simulink model "MPC"  (R2024b)
settings: Solver=ode4  StartTime=0.0  StopTime=tsim  FixedStep=baseRate  RelTol=1e-6  AbsTol=1e-6
values from neighbouring files (symbols this model uses):
  C = [cos(theta), -sin(theta) ... (first row only)    [Run_Initializer.m]    (also in plotBatch.m = quat2Rotm(q','scalarFirst'))
  camera_FOV = 40*d2r    (= 0.698131700798)    [Run_Initializer.m]
  camera_offset = [0.145, 0.087]'    [Run_Initializer.m]
  docking_face = [0 1]'    [Run_Initializer.m]
  docking_offset = [0 0 0]'    [Run_Initializer.m]
  eta = 0.7    [Run_Initializer.m]
  F_t = [kron(eye(N_h),  [zeros(2,3), eye(2), zeros(2,4)]) ... (first row only)    [Run_Initializer.m]
  f_t = [kron(ones(N_h, 1), [xLength yLength]' - edge_buffer) ... (first row only)    [Run_Initializer.m]
  F_u = [kron(eye(N_h),  [eye(3), zeros(3,6)]) ... (first row only)    [Run_Initializer.m]
  f_u = kron(ones(2*N_h, 1), u_max')    [Run_Initializer.m]
  F_v = [kron(eye(N_h),  [zeros(1,5), 1, zeros(1,3)]) ... (first row only)    [Run_Initializer.m]
  gamma = 0.95    [Run_Initializer.m]
  Gamma1_el = 0.12    [Run_Initializer.m]
  Gamma1_sh = 0.005    [Run_Initializer.m]
  Gamma1_wr = 0.025    [Run_Initializer.m]
  Gamma2_el = 5    [Run_Initializer.m]
  Gamma2_sh = 5    [Run_Initializer.m]
  Gamma2_wr = 5    [Run_Initializer.m]
  Gamma3_el = 10    [Run_Initializer.m]
  Gamma3_sh = 40    [Run_Initializer.m]
  Gamma3_wr = 40    [Run_Initializer.m]
  Gamma4_el = 0.039    [Run_Initializer.m]
  Gamma4_sh = 0.015    [Run_Initializer.m]
  Gamma4_wr = 0.029    [Run_Initializer.m]
  Gamma5_el = 800    [Run_Initializer.m]
  Gamma5_sh = 800    [Run_Initializer.m]
  Gamma5_wr = 800    [Run_Initializer.m]
  Gamma6_el = 0.000001    (= 1e-06)    [Run_Initializer.m]
  Gamma6_sh = 0.005    [Run_Initializer.m]
  Gamma6_wr = 0.02    [Run_Initializer.m]
  H = kron(eye(N_h), [R, zeros(3,6); zeros(6,3), Q])    [Run_Initializer.m]
  IBLACK = 0.1996    [unpackData.m]
  IRED = 0.1982    [unpackData.m]
  J = sum(wp*posErr + wt*angErr)    [find_transformation.m]
  Kd_elarm = 0.8    [Run_Initializer.m]
  Kd_sharm = 1.0    (= 1)    [Run_Initializer.m]
  Kd_wrarm = 0.6    [Run_Initializer.m]
  Kp_elarm = 1.2    [Run_Initializer.m]
  Kp_sharm = 1.5    [Run_Initializer.m]
  Kp_wrarm = 1.0    (= 1)    [Run_Initializer.m]
  m = m + 5    (= 4)    [unpackData.m]
  M = diag([1/m; 1/m; 1/I])    [unpackData.m]
  maxd = [d1 ... (first row only)    [Run_Initializer.m]
  mBLACK = 11.3620    (= 11.362)    [unpackData.m]
  mRED = 11.2970    (= 11.297)    [unpackData.m]
  N = size(rel,1)    [plotBatch.m]    (also in unpackData.m = 0)
  p = [0 obj.pos(k,:)]    [SparseState6DOF.m]
  PDQ = blkdiag(20*eye(3),eye(3), 20*eye(3),eye(3))    [Run_Initializer.m]
  PQ = blkdiag(20*eye(6),eye(6))    [Run_Initializer.m]
  PR = blkdiag(20*eye(3), eye(6), 0.0001*eye(3))    [Run_Initializer.m]
  PWMFreq = 5    [Run_Initializer.m]
  Q = diag([100 100 100 300 300 300])    [Run_Initializer.m]    (also in unpackData.m = blkdiag(0.0001*eye(2), 0.00001))
  R = diag([200 200 200])    [Run_Initializer.m]    (also in plotBatch.m = C3(yaw); unpackData.m = diag([6;6;6]))
  r_hold_obs = 1.1*sqrt(2)*0.3.*[1 1]    [Run_Initializer.m]
  r_hold_tar_min = [0.8; (0.3+0.05)]    [Run_Initializer.m]
  rho = 0.98    [Run_Initializer.m]
  T_d = 2    [Run_Initializer.m]
  T_max = 0.15    [Run_Initializer.m]
  Tz_lim_elarm = .1    (= 0.1)    [Run_Initializer.m]
  Tz_lim_sharm = .1    (= 0.1)    [Run_Initializer.m]
  Tz_lim_wrarm = .1    (= 0.1)    [Run_Initializer.m]
  use_LOS_constr = 1    [Run_Initializer.m]
  use_table_constr = 1    [Run_Initializer.m]
  x_BLACK_0 = [(1/3)*xLength (1/3)*yLength-0.2 280*d2r 0.01 0.005 1.88*d2r]'    [Run_Initializer.m]
  x_BLUE_0 = [0 0 0 0 0 0]'    [Run_Initializer.m]
  zeta = 10*d2r    (= 0.174532925199)    [Run_Initializer.m]
undefined symbols (not defined in the file or in its folder): a1, a2, a3, alpha, alpha_m, alpha_t, alphas, alphas_t, alphat, Am, b, b0, b1, b2, b3, baseRate, Bm, c, c1, c1t, c2, c2t, Cm, d, dataRate, DiscIntNeverNeededParam, Dm, drop_states_ARM, drop_states_BLACK, drop_states_BLUE, drop_states_RED, epsilon, epsilont, F_black_X_nominal, F_black_Y_nominal, F_blue_X_nominal, F_blue_Y_nominal, F_max, F_red_X_nominal, F_red_Y_nominal, F_thrusters_BLACK, F_thrusters_BLUE, F_thrusters_RED, gamma_I, gamma_I_t, gamma_P, gamma_P_t, home_states_BLACK, home_states_BLUE, home_states_RED, IBLUE, IDIST, IEE, init_states_BLACK, init_states_BLUE, init_states_RED, IPROX, k, K, k1 ... (+62)
libraries: simulink x33, nvidiaSharedBlocks x13, slpidlib x6, MainLibrary x5, dspsigops x3, dspinverses x3, nvidiaIMUSensorslib x1
(part 12 of 12)

== matlab function MPC/Thruster Control Code/Change BLACK Behavior/Calculate Duty Cycle/Generate Initial Guess/MATLAB Function ==
  data: H output; thruster_dist2CG_BLACK parameter; F_thrusters_BLACK parameter
function H = MakeH(thruster_dist2CG_BLACK,F_thrusters_BLACK)

    Vec1 = [ -1
             -1
              0 
              0
              1
              1
              0
              0 ];
          
    Vec2 = [  0
              0
              1
              1
              0
              0
             -1
             -1 ];
         
    Vec3 = thruster_dist2CG_BLACK./1000;
    
    Mat1 = [Vec1, Vec2, Vec3]';
    
    Mat2 = diag((F_thrusters_BLACK./2));
    
    H    = Mat1*Mat2;

end

== matlab function MPC/PhaseSpace Filter Code/Subsystem3/Subsystem/MATLAB Function1 ==
  data: u input; y output; uprev input
function y = fcn(u, uprev)
    if sum(abs(u-uprev)) < 10^-10
        y = NaN(3,1);
    else
        y = [u(1:2);unwrap(u(3))];
    end
end

== matlab function MPC/Thruster Control Code/Change BLACK Behavior/Calculate Duty Cycle/MATLAB Function1 ==
  data: ThrustPer_Final output; ThrustPer input; PWMFreq parameter
function ThrustPer_Final  = ThrusterSat(ThrustPer, PWMFreq)

    ValveTime       = 0.007;
    TControl        = 1/PWMFreq;

    ThrustPer_Final = zeros(8,1);
    
    if max(ThrustPer) > 1
        ThrustPer_Sat = ThrustPer/max(ThrustPer);
    else
        ThrustPer_Sat = ThrustPer;
    end
    
    for i = 1:8
        if ThrustPer_Sat(i) > ValveTime/TControl 
            ThrustPer_Final(i) = ThrustPer_Sat(i);
        else
            %ThrustPer_Final(i) = 0;
        end
    end


end

== matlab function MPC/PhaseSpace Filter Code/Subsystem1/Subsystem/MATLAB Function1 ==
  data: u input; y output; uprev input
function y = fcn(u, uprev)
    if sum(abs(u-uprev)) < 10^-10
        y = NaN(3,1);
    else
        y = [u(1:2);unwrap(u(3))];
    end
end

== matlab function MPC/4 - Control/Default PD Control (RED)/Calculate Error/MATLAB Function ==
  data: Rz_path input; Rz_error output; Rz_measured input
function Rz_error = SmoothAngularDifference(Rz_path, Rz_measured)

    Rz_error = mod(Rz_measured-Rz_path+pi, 2*pi)-pi;


end

== matlab function MPC/4 - Control/Disable Thrusters (BLACK)/MATLAB Function ==
  data: u input; y output
function y = fcn(u)
    y = zeros(6,1);
end

== matlab function MPC/Model Predictive Control/Model Predictive Control/Compute Target Trajectory ==
  data: r_hold_tar input; z_RED input; z_BLACK input; docking input; docking_face parameter; z_t output; docking_offset parameter
% Compute docking position over the horizon
function z_t  = fcn(r_hold_tar, z_RED, z_BLACK, docking, docking_face, docking_offset)

% Define horizon length
N_h = 15;

% Pre-allocate target trajectory vector
z_t = zeros(9*N_h,1);

% Iterate over the horizon
for j = 1:N_h
    pos = 9*(j-1)+1;
    % Compute 2D z-axis rotation matrix representing the targets attitude
    R = rotz(z_BLACK(pos+5));

    % Compute the docking position in the global frame relative to the target
    r_dock = R*(r_hold_tar(2).*docking_face + docking_offset(1:2));

    if docking
        theta_star = z_BLACK(pos+5) + docking_offset(3)-pi/2;
    else
        theta_star = rotateToFace(z_RED(pos+5), z_BLACK(pos+3:pos+4)-z_RED(pos+3:pos+4)) + docking_offset(3);
    end

    % Store required attitude and position for docking
    z_t(pos+3:pos+4) = z_BLACK(pos+3:pos+4) + r_dock;
    z_t(pos+5) = theta_star;
end

end

%% Functions

function C = rotz(theta)
    C = [cos(theta) -sin(theta); sin(theta) cos(theta)];
end

function theta_des = rotateToFace(theta, r)
    theta_des = theta + wrapToPi(atan2(r(2),r(1)) - theta);
end

== matlab function MPC/Model Predictive Control/Model Predictive Control/Dynamic Target Collision Constraint ==
  data: r_hold_tar input; z_BLACK input; F_h output; z_RED input; f_h output
function [F_h, f_h] = fcn(r_hold_tar, z_BLACK, z_RED)

% Define horizon length
N_h = 15;

% Define shape matrix
S = diag(r_hold_tar.^-2);

% Pre-allocate expansion point position vector over the horizon
r_0_bar = zeros(9*N_h,1);

% Pre-allocate D matrix
F_h = zeros(N_h, 9*N_h);
f_h = zeros(N_h,1);

% Iterate over the horizon
for j = 1:N_h
    pos = 9*(j-1)+1;
    
    % Extract target & chaser positions, and target attitude
    r_tar = z_BLACK(pos+3:pos+4);
    r_chs = z_RED(pos+3:pos+4);
    theta_tar = z_BLACK(pos+5);

    % Compute target -> chaser unit vector
    u_tc = (r_chs-r_tar)/norm(r_chs-r_tar);

    % Compute target body-fixed -> inertial rotation matrix
    R = [cos(theta_tar) -sin(theta_tar); 
         sin(theta_tar) cos(theta_tar)];

    % Compute angle between target-chaser vector and target body-fixed
    % x-axis in inertial frame
    theta_e = acos(u_tc'*(R*[1; 0]));

    % Extract semi-(major/minor) axes
    [a_e, b_e] = deal(r_hold_tar(1), r_hold_tar(2));

    % Compute ellipse radius at current angle
    r_e = a_e*b_e/sqrt((a_e*sin(theta_e))^2 + (b_e*cos(theta_e))^2);

    % Compute expansion point position
    r_0 = r_tar + r_e.*u_tc;

    % Store expansion point positions in respective vector
    r_0_bar(pos+3:pos+4) = r_0;

    % Compute E matrix
    E = (r_0-r_tar)'*(R*S*R');

    row = j;
    col = 3+9*(j-1)+1;

    F_hj = -2.*E;
    f_hj = -1-E*(r_0+r_tar);

    F_h(row,col:col+1) = F_hj;
    f_h(row,1) = f_hj;

end

end

== matlab function MPC/4 - Control/Default PD Control (RED)/CSMC/MATLAB Function ==
  data: phi input; u output; alpha parameter
function u = fcn(phi, alpha)



u = sign(phi)*(abs(phi)^(alpha/(2 - alpha)));

== matlab function MPC/4 - Control/Default PD Control (RED)/CSMC/MATLAB Function1 ==
  data: q2 input; u output; k1 parameter; alpha parameter
function u = fcn(q2,k1, alpha)

u = sign(k1*q2)*(abs(k1*q2)^alpha);

== matlab function MPC/4 - Control/Default PD Control (RED)/SAC/Ideal Plant Model3/MATLAB Function ==
  data: x output; u input; y output; t output; dx output; dy output; dt output
function [x,y,t,dx,dy,dt] = fcn(u)
x = u(1);
y = u(2);
t = u(3);
dx = u(4);
dy = u(5);
dt = u(6);
end

== matlab function MPC/4 - Control/Default PD Control (RED)/SAC/SAC_CTL/Position/Storage/MATLAB Function ==
  data: u input; y1 output; y2 output; y3 output; y4 output
function [y1,y2,y3,y4] = fcn(u)
y1 = u(1);
y2 = u(2);
y3 = u(3);
y4 = u(4);
end

== matlab function MPC/4 - Control/Default PD Control (RED)/SAC/SAC_CTL/Position/Storage/MATLAB Function2 ==
  data: u input; y1 output; y2 output; y3 output; y4 output
function [y1,y2,y3,y4] = fcn(u)
y1 = u(1);
y2 = u(2);
y3 = u(3);
y4 = u(4);
end

== matlab function MPC/Model Predictive Control/Model Predictive Control/Obstacle Collision Constraint ==
  data: z_BLUE input; F_c output; z_RED input; f_c output; r_hold_obs parameter; platformSelection parameter
function [F_c, f_c] = fcn(z_BLUE, z_RED, r_hold_obs, platformSelection)

% Define horizon length
N_h = 15;

% Define shape matrix
S = diag(r_hold_obs.^-2);

% Pre-allocate expansion point position vector over the horizon
r_0_bar = zeros(9*N_h,1);

% Pre-allocate D matrix
F_c = zeros(N_h, 9*N_h);
f_c = zeros(N_h,1);

if platformSelection >= 6 && platformSelection <= 11
    
    % Iterate over the horizon
    for j = 1:N_h
        pos = 9*(j-1)+1;
        
        % Extract target & chaser positions, and target attitude
        r_tar = z_BLUE(pos+3:pos+4);
        r_chs = z_RED(pos+3:pos+4);
        theta_tar = z_BLUE(pos+5);
    
        % Compute target -> chaser unit vector
        u_tc = (r_chs-r_tar)/norm(r_chs-r_tar);
    
        % Compute target body-fixed -> inertial rotation matrix
        R = [cos(theta_tar) -sin(theta_tar); 
             sin(theta_tar) cos(theta_tar)];
    
        % Compute angle between target-chaser vector and target body-fixed
        % x-axis in inertial frame
        theta_e = acos(u_tc'*(R*[1; 0]));
    
        % Extract semi-(major/minor) axes
        [a_e, b_e] = deal(r_hold_obs(1), r_hold_obs(2));
    
        % Compute ellipse radius at current angle
        r_e = a_e*b_e/sqrt((a_e*sin(theta_e))^2 + (b_e*cos(theta_e))^2);
    
        % Compute expansion point position
        r_0 = r_tar + r_e.*u_tc;
    
        % Store expansion point positions in respective vector
        r_0_bar(pos+3:pos+4) = r_0;
    
        % Compute E matrix
        E = (r_0-r_tar)'*(R*S*R');
    
        row = j;
        col = 3+9*(j-1)+1;
    
        F_hj = -2.*E;
        f_hj = -1-E*(r_0+r_tar);
    
        F_c(row,col:col+1) = F_hj;
        f_c(row,1) = f_hj;
    
    end
end

end

== matlab function MPC/Model Predictive Control/Model Predictive Control/Shift Optimization Variable ==
  data: z input; z_0 output
function z_0 = fcn(z)

% Shift reference trajectory by dropping first control input and state,
% set last control input as zeros and duplicate last state
z_0 = [z(9+1:end); zeros(3,1); z(end-5:end)];

end

== matlab function MPC/4 - Control/Default PD Control (RED)/Diff/Hough Control/MATLAB Function2 ==
  data: Oy output; z input; Ox output
function [Oy, Ox]   = C3( z )
%C3 gives the rotation matrix about the z-axis for an angle 'z'
%   z - the angle about the z-axis which you rotate
%   A - the rotation matrix

Ox = [cos(z) sin(z); -sin(z) cos(z)]*[1;0];
Oy = [cos(z) sin(z); -sin(z) cos(z)]*[0;1];
end

== matlab function MPC/4 - Control/Default PD Control (RED)/Diff/Hough Control/MATLAB Function3 ==
  data: z input; Ox output
function Ox    = C3( z )
%C3 gives the rotation matrix about the z-axis for an angle 'z'
%   z - the angle about the z-axis which you rotate
%   A - the rotation matrix

Ox = [cos(z) sin(z); -sin(z) cos(z)]*[1;0];
end

== matlab function MPC/4 - Control/Default PD Control (RED)/Diff/Hough Control/MATLAB Function4 ==
  data: Oy input; e_out output; e_in input
function e_out = fcn(Oy, e_in)

a = sign(Oy'*e_in);
e_out = -a*norm(e_in);

== matlab function MPC/4 - Control/Default PD Control (RED)/MATLAB Function ==
  data: u input; y output
function y = fcn(u)

y = u(1:3);

== matlab function MPC/Thruster Control Code/Change BLACK Behavior/Calculate Duty Cycle/MATLAB Function5 ==
  data: H_final output; u_desired input; duty_cycles output; x0 input; thruster_dist2CG_BLACK parameter; F_black_X_nominal parameter; F_black_Y_nominal parameter; max_iters parameter; tol parameter
function [H_final,duty_cycles] = optimize_duty_cycle_with_decay(u_desired, x0, thruster_dist2CG_BLACK, F_black_X_nominal, F_black_Y_nominal, max_iters, tol)
    % Optimizes thruster duty cycles with decay factor updates
    %
    % Inputs:
    %   u_desired - Desired force and torque vector [Fx; Fy; M] (3x1)
    %   x0 - Initial guess for duty cycles (vector, 8x1)
    %   max_iters - Maximum number of iterations for convergence
    %   tol - Convergence tolerance for duty cycles
    %   thruster_dist2CG_BLACK - Distances of thrusters from CG (vector, mm)
    %   F_red_X_nominal - Nominal X thruster force (scalar, N)
    %   F_red_Y_nominal - Nominal Y thruster force (scalar, N)
    %
    % Outputs:
    %   duty_cycles - Optimal duty cycles for each thruster (vector, 8x1)

    % Initialization
    num_thrusters = length(x0);
    duty_cycles = x0; % Start with the initial guess
    thrust_decay_factor = 1; % Initial decay factor
    prev_duty_cycles = duty_cycles + 2 * tol; % Ensure loop starts

    % Iterative optimization process
    for iter = 1:max_iters
        % Update H matrix based on the current decay factor
        H = MakeHWithDecay(thruster_dist2CG_BLACK, F_black_X_nominal, thrust_decay_factor, F_black_Y_nominal);
        
        % Define quadratic programming problem
        Q = 2 * (H' * H); % Quadratic term
        c = -2 * (H' * u_desired); % Linear term
        lb = zeros(num_thrusters, 1); % Lower bounds
        ub = ones(num_thrusters, 1); % Upper bounds
        options = optimoptions('quadprog', 'Display', 'off', 'Algorithm', 'active-set', 'MaxIterations', 5);
        
        % Solve for optimal duty cycles
        [duty_cycles, ~, ~] = quadprog(Q, c, [], [], [], [], lb, ub, duty_cycles, options);
        
        % Update decay factor based on the current duty cycles
        [thrust_decay_factor, ~] = check_thrust_decay(duty_cycles);
                
        % Check convergence criteria
        if norm(duty_cycles - prev_duty_cycles, Inf) < tol
            H_final = MakeHWithDecayRecalculateForce(thruster_dist2CG_BLACK, F_black_X_nominal, thrust_decay_factor, F_black_Y_nominal);
            return;
        end
            
        
        % Update for next iteration
        prev_duty_cycles = duty_cycles;
    end
    
    H_final = MakeHWithDecayRecalculateForce(thruster_dist2CG_BLACK, F_black_X_nominal, thrust_decay_factor, F_black_Y_nominal);
   

end

function H = MakeHWithDecay(thruster_dist2CG, F_X_nominal, thrust_decay_factor, F_Y_nominal)
    % Constructs the H matrix with thrust decay adjustments
    %
    % Inputs:
    %   thruster_dist2CG - Distances of thrusters from CG (vector, mm)
    %   F_X_nominal - Nominal X thruster force (scalar, N)
    %   thrust_decay_factor - Decay factor for thrust (scalar)
    %   F_Y_nominal - Nominal Y thruster force (scalar, N)
    %
    % Output:
    %   H - H matrix for optimization (3x8)

    % Adjust thruster distances (convert to meters)
    adjusted_thruster_dist2CG = thruster_dist2CG / 1000;

    % Define thruster contribution vectors
    Vec1 = [-1; -1;  0;  0;  1;  1;  0;  0]; % X-component
    Vec2 = [ 0;  0;  1;  1;  0;  0; -1; -1]; % Y-component
    Vec3 = adjusted_thruster_dist2CG;        % Moment arm (Z)

    % Combine vectors into the H matrix structure
    Mat1 = [Vec1, Vec2, Vec3]';
    
    % Adjust thruster forces with decay factor
    F_thrusters = [F_X_nominal; F_X_nominal; F_Y_nominal; F_Y_nominal; 
                   F_X_nominal; F_X_nominal; F_Y_nominal; F_Y_nominal] * thrust_decay_factor;

    % Scale forces for H matrix
    Mat2 = diag(F_thrusters / 2);

    % Compute final H matrix
    H = Mat1 * Mat2;
end

function H = MakeHWithDecayRecalculateForce(thruster_dist2CG, F_X_nominal, thrust_decay_factor, F_Y_nominal)
    % Constructs the H matrix with thrust decay adjustments
    %
    % Inputs:
    %   thruster_dist2CG - Distances of thrusters from CG (vector, mm)
    %   F_X_nominal - Nominal X thruster force (scalar, N)
    %   thrust_decay_factor - Decay factor for thrust (scalar)
    %   F_Y_nominal - Nominal Y thruster force (scalar, N)
    %
    % Output:
    %   H - H matrix for optimization (3x8)

    % Adjust thruster distances (convert to meters)
    adjusted_thruster_dist2CG = thruster_dist2CG / 1000;

    % Define thruster contribution vectors
    Vec1 = [-1; -1;  0;  0;  1;  1;  0;  0]; % X-component
    Vec2 = [ 0;  0;  1;  1;  0;  0; -1; -1]; % Y-component
    Vec3 = adjusted_thruster_dist2CG;        % Moment arm (Z)

    % Combine vectors into the H matrix structure
    Mat1 = [Vec1, Vec2, Vec3]';
    
    % Adjust thruster forces with decay factor
    F_thrusters = [F_X_nominal; F_X_nominal; F_Y_nominal; F_Y_nominal; 
                   F_X_nominal; F_X_nominal; F_Y_nominal; F_Y_nominal] * thrust_decay_factor;

    % Scale forces for H matrix
    Mat2 = diag(F_thrusters);

    % Compute final H matrix
    H = Mat1 * Mat2;
end

function [thrust_decay_factor, count] = check_thrust_decay(PWMs)
    % Updates the thrust decay factor based on current duty cycles
    %
    % Inputs:
    %   PWMs - Current duty cycle values (vector)
    %
    % Outputs:
    %   thrust_decay_factor - Updated decay factor (scalar)
    %   count - Number of active thrusters (scalar)

    % Normalize PWMs if necessary
    if max(PWMs) > 1
        PWMs = PWMs / max(PWMs);
    end

    % Count active thrusters
    count = sum(PWMs > 0);
    
    % Compute average duty cycle for active thrusters
    average_duty_cycle_per_thruster = sum(max(PWMs, 0)) / max(count, 1);

    % Update thrust decay factor based on average duty cycle
    if average_duty_cycle_per_thruster < 0.3 || count == 0
        thrust_decay_factor = 1;
    else
        thrust_decay_factor = max(0.6 - 2 * average_duty_cycle_per_thruster + 1, 0.5);
    end
end

== matlab function MPC/Thruster Control Code/Change BLACK Behavior/Calculate Duty Cycle/Rotate Forces to Inertial/Create Rotation Matrix ==
  data: Rz input; C_Ib output
function C_Ib = RotateFrame(Rz)

C_bI = [  cos(Rz) sin(Rz)
         -sin(Rz) cos(Rz) ];

C_Ib = inv(C_bI);

end

== matlab function MPC/Data Logger Subsystem/Subsystem1/MATLAB Function ==
  data: u input; y output
function y = fcn(u)

if anynan(u)
    y = -1*ones(size(u));
else
    y = u;
end
end

== matlab function MPC/4 - Control/Default PD Control (BLACK)/Calculate Error/MATLAB Function ==
  data: Rz_path input; Rz_error output; Rz_measured input
function Rz_error = SmoothAngularDifference(Rz_path, Rz_measured)

    Rz_error = mod(Rz_measured-Rz_path+pi, 2*pi)-pi;


end

== matlab function MPC/Thruster Control Code/Change BLACK Behavior/Rotate Forces to Body/Create Rotation Matrix ==
  data: Rz input; C_bI output
function C_bI = RotateFrame(Rz)

C_bI = [  cos(Rz) sin(Rz)
         -sin(Rz) cos(Rz) ];

end

== matlab function MPC/Thruster Control Code/Change BLUE Behavior/Calculate Duty Cycle/Generate Initial Guess/MATLAB Function ==
  data: H output; thruster_dist2CG_BLUE parameter; F_thrusters_BLUE parameter
function H = MakeH(thruster_dist2CG_BLUE,F_thrusters_BLUE)

    Vec1 = [ -1
             -1
              0 
              0
              1
              1
              0
              0 ];
          
    Vec2 = [  0
              0
              1
              1
              0
              0
             -1
             -1 ];
         
    Vec3 = thruster_dist2CG_BLUE./1000;
    
    Mat1 = [Vec1, Vec2, Vec3]';
    
    Mat2 = diag((F_thrusters_BLUE./2));
    
    H    = Mat1*Mat2;

end

== matlab function MPC/Thruster Control Code/Change BLUE Behavior/Calculate Duty Cycle/MATLAB Function1 ==
  data: ThrustPer_Final output; ThrustPer input; PWMFreq parameter
function ThrustPer_Final  = ThrusterSat(ThrustPer, PWMFreq)

    ValveTime       = 0.007;
    TControl        = 1/PWMFreq;

    ThrustPer_Final = zeros(8,1);
    
    if max(ThrustPer) > 1
        ThrustPer_Sat = ThrustPer/max(ThrustPer);
    else
        ThrustPer_Sat = ThrustPer;
    end
    
    for i = 1:8
        if ThrustPer_Sat(i) > ValveTime/TControl 
            ThrustPer_Final(i) = ThrustPer_Sat(i);
        else
            ThrustPer_Final(i) = 0;
        end
    end


end

== matlab function MPC/Thruster Control Code/Change BLUE Behavior/Calculate Duty Cycle/MATLAB Function5 ==
  data: H_final output; u_desired input; duty_cycles output; x0 input; thruster_dist2CG_BLUE parameter; F_blue_X_nominal parameter; F_blue_Y_nominal parameter; max_iters parameter; tol parameter
function [H_final,duty_cycles] = optimize_duty_cycle_with_decay(u_desired, x0, thruster_dist2CG_BLUE, F_blue_X_nominal, F_blue_Y_nominal, max_iters, tol)
    % Optimizes thruster duty cycles with decay factor updates
    %
    % Inputs:
    %   u_desired - Desired force and torque vector [Fx; Fy; M] (3x1)
    %   x0 - Initial guess for duty cycles (vector, 8x1)
    %   max_iters - Maximum number of iterations for convergence
    %   tol - Convergence tolerance for duty cycles
    %   thruster_dist2CG_BLUE - Distances of thrusters from CG (vector, mm)
    %   F_red_X_nominal - Nominal X thruster force (scalar, N)
    %   F_red_Y_nominal - Nominal Y thruster force (scalar, N)
    %
    % Outputs:
    %   duty_cycles - Optimal duty cycles for each thruster (vector, 8x1)

    % Initialization
    if anynan(u_desired)
        disp('ohhh noooo!!!')
    end

    num_thrusters = length(x0);
    duty_cycles = x0; % Start with the initial guess
    thrust_decay_factor = 1; % Initial decay factor
    prev_duty_cycles = duty_cycles + 2 * tol; % Ensure loop starts

    % Iterative optimization process
    for iter = 1:max_iters
        % Update H matrix based on the current decay factor
        H = MakeHWithDecay(thruster_dist2CG_BLUE, F_blue_X_nominal, thrust_decay_factor, F_blue_Y_nominal);
        
        % Define quadratic programming problem
        Q = 2 * (H' * H); % Quadratic term
        c = -2 * (H' * u_desired); % Linear term
        lb = zeros(num_thrusters, 1); % Lower bounds
        ub = ones(num_thrusters, 1); % Upper bounds
        options = optimoptions('quadprog', 'Display', 'off', 'Algorithm', 'active-set', 'MaxIterations', 5);
        
        % Solve for optimal duty cycles
        [duty_cycles, ~, ~] = quadprog(Q, c, [], [], [], [], lb, ub, duty_cycles, options);
        
        % Update decay factor based on the current duty cycles
        [thrust_decay_factor, ~] = check_thrust_decay(duty_cycles);
                
        % Check convergence criteria
        if norm(duty_cycles - prev_duty_cycles, Inf) < tol
            H_final = MakeHWithDecayRecalculateForce(thruster_dist2CG_BLUE, F_blue_X_nominal, thrust_decay_factor, F_blue_Y_nominal);
            return;
        end
            
        
        % Update for next iteration
        prev_duty_cycles = duty_cycles;
    end
    
    H_final = MakeHWithDecayRecalculateForce(thruster_dist2CG_BLUE, F_blue_X_nominal, thrust_decay_factor, F_blue_Y_nominal);
   

end

function H = MakeHWithDecay(thruster_dist2CG, F_X_nominal, thrust_decay_factor, F_Y_nominal)
    % Constructs the H matrix with thrust decay adjustments
    %
    % Inputs:
    %   thruster_dist2CG - Distances of thrusters from CG (vector, mm)
    %   F_X_nominal - Nominal X thruster force (scalar, N)
    %   thrust_decay_factor - Decay factor for thrust (scalar)
    %   F_Y_nominal - Nominal Y thruster force (scalar, N)
    %
    % Output:
    %   H - H matrix for optimization (3x8)

    % Adjust thruster distances (convert to meters)
    adjusted_thruster_dist2CG = thruster_dist2CG / 1000;

    % Define thruster contribution vectors
    Vec1 = [-1; -1;  0;  0;  1;  1;  0;  0]; % X-component
    Vec2 = [ 0;  0;  1;  1;  0;  0; -1; -1]; % Y-component
    Vec3 = adjusted_thruster_dist2CG;        % Moment arm (Z)

    % Combine vectors into the H matrix structure
    Mat1 = [Vec1, Vec2, Vec3]';
    
    % Adjust thruster forces with decay factor
    F_thrusters = [F_X_nominal; F_X_nominal; F_Y_nominal; F_Y_nominal; 
                   F_X_nominal; F_X_nominal; F_Y_nominal; F_Y_nominal] * thrust_decay_factor;

    % Scale forces for H matrix
    Mat2 = diag(F_thrusters / 2);

    % Compute final H matrix
    H = Mat1 * Mat2;
end

function H = MakeHWithDecayRecalculateForce(thruster_dist2CG, F_X_nominal, thrust_decay_factor, F_Y_nominal)
    % Constructs the H matrix with thrust decay adjustments
    %
    % Inputs:
    %   thruster_dist2CG - Distances of thrusters from CG (vector, mm)
    %   F_X_nominal - Nominal X thruster force (scalar, N)
    %   thrust_decay_factor - Decay factor for thrust (scalar)
    %   F_Y_nominal - Nominal Y thruster force (scalar, N)
    %
    % Output:
    %   H - H matrix for optimization (3x8)

    % Adjust thruster distances (convert to meters)
    adjusted_thruster_dist2CG = thruster_dist2CG / 1000;

    % Define thruster contribution vectors
    Vec1 = [-1; -1;  0;  0;  1;  1;  0;  0]; % X-component
    Vec2 = [ 0;  0;  1;  1;  0;  0; -1; -1]; % Y-component
    Vec3 = adjusted_thruster_dist2CG;        % Moment arm (Z)

    % Combine vectors into the H matrix structure
    Mat1 = [Vec1, Vec2, Vec3]';
    
    % Adjust thruster forces with decay factor
    F_thrusters = [F_X_nominal; F_X_nominal; F_Y_nominal; F_Y_nominal; 
                   F_X_nominal; F_X_nominal; F_Y_nominal; F_Y_nominal] * thrust_decay_factor;

    % Scale forces for H matrix
    Mat2 = diag(F_thrusters);

    % Compute final H matrix
    H = Mat1 * Mat2;
end

function [thrust_decay_factor, count] = check_thrust_decay(PWMs)
    % Updates the thrust decay factor based on current duty cycles
    %
    % Inputs:
    %   PWMs - Current duty cycle values (vector)
    %
    % Outputs:
    %   thrust_decay_factor - Updated decay factor (scalar)
    %   count - Number of active thrusters (scalar)

    % Normalize PWMs if necessary
    if max(PWMs) > 1
        PWMs = PWMs / max(PWMs);
    end

    % Count active thrusters
    count = sum(PWMs > 0);
    
    % Compute average duty cycle for active thrusters
    average_duty_cycle_per_thruster = sum(max(PWMs, 0)) / max(count, 1);

    % Update thrust decay factor based on average duty cycle
    if average_duty_cycle_per_thruster < 0.3 || count == 0
        thrust_decay_factor = 1;
    else
        thrust_decay_factor = max(0.6 - 2 * average_duty_cycle_per_thruster + 1, 0.5);
    end
end

== matlab function MPC/4 - Control/Default LQR Control (RED)/Calculate Error/MATLAB Function ==
  data: Rz_path input; Rz_error output; Rz_measured input
function Rz_error = SmoothAngularDifference(Rz_path, Rz_measured)

    Rz_error = mod(Rz_measured-Rz_path+pi, 2*pi)-pi;


end

== matlab function MPC/4 - Control/Default PD Control (RED)/SAC/SAC_CTL/Position/Storage/MATLAB Function1 ==
  data: u input; y1 output; y2 output; y3 output; y4 output
function [y1,y2,y3,y4] = fcn(u)
y1 = u(1);
y2 = u(2);
y3 = u(3);
y4 = u(4);
end

== matlab function MPC/Thruster Control Code/Change BLUE Behavior/Calculate Duty Cycle/Rotate Forces to Inertial/Create Rotation Matrix ==
  data: Rz input; C_Ib output
function C_Ib = RotateFrame(Rz)

C_bI = [  cos(Rz) sin(Rz)
         -sin(Rz) cos(Rz) ];

C_Ib = inv(C_bI);

end

== matlab function MPC/Thruster Control Code/Change BLUE Behavior/Rotate Forces to Body/Create Rotation Matrix ==
  data: Rz input; C_bI output
function C_bI = RotateFrame(Rz)

C_bI = [  cos(Rz) sin(Rz)
         -sin(Rz) cos(Rz) ];

end

== matlab function MPC/Thruster Control Code/Change RED Behavior/Calculate Duty Cycle/Generate Initial Guess/MATLAB Function ==
  data: H output; thruster_dist2CG_RED parameter; F_thrusters_RED parameter
function H = MakeH(thruster_dist2CG_RED,F_thrusters_RED)

    Vec1 = [ -1
             -1
              0 
              0
              1
              1
              0
              0 ];
          
    Vec2 = [  0
              0
              1
              1
              0
              0
             -1
             -1 ];
         
    Vec3 = thruster_dist2CG_RED./1000;
    
    Mat1 = [Vec1, Vec2, Vec3]';
    
    Mat2 = diag((F_thrusters_RED./2));
    
    H    = Mat1*Mat2;

end

== matlab function MPC/Thruster Control Code/Change RED Behavior/Calculate Duty Cycle/MATLAB Function5 ==
  data: H_final output; u_desired input; duty_cycles output; x0 input; thruster_dist2CG_RED parameter; F_red_X_nominal parameter; F_red_Y_nominal parameter; max_iters parameter; tol parameter
function [H_final,duty_cycles] = optimize_duty_cycle_with_decay(u_desired, x0, thruster_dist2CG_RED, F_red_X_nominal, F_red_Y_nominal, max_iters, tol)
    % Optimizes thruster duty cycles with decay factor updates
    %
    % Inputs:
    %   u_desired - Desired force and torque vector [Fx; Fy; M] (3x1)
    %   x0 - Initial guess for duty cycles (vector, 8x1)
    %   max_iters - Maximum number of iterations for convergence
    %   tol - Convergence tolerance for duty cycles
    %   thruster_dist2CG_RED - Distances of thrusters from CG (vector, mm)
    %   F_red_X_nominal - Nominal X thruster force (scalar, N)
    %   F_red_Y_nominal - Nominal Y thruster force (scalar, N)
    %
    % Outputs:
    %   duty_cycles - Optimal duty cycles for each thruster (vector, 8x1)

    % Initialization
    num_thrusters = length(x0);
    duty_cycles = x0; % Start with the initial guess
    thrust_decay_factor = 1; % Initial decay factor
    prev_duty_cycles = duty_cycles + 2 * tol; % Ensure loop starts

    % Iterative optimization process
    for iter = 1:max_iters
        % Update H matrix based on the current decay factor
        H = MakeHWithDecay(thruster_dist2CG_RED, F_red_X_nominal, thrust_decay_factor, F_red_Y_nominal);
        
        % Define quadratic programming problem
        Q = 2 * (H' * H); % Quadratic term
        c = -2 * (H' * u_desired); % Linear term
        lb = zeros(num_thrusters, 1); % Lower bounds
        ub = ones(num_thrusters, 1); % Upper bounds
        options = optimoptions('quadprog', 'Display', 'off', 'Algorithm', 'active-set', 'MaxIterations', 5);
        
        % Solve for optimal duty cycles
        [duty_cycles, ~, ~] = quadprog(Q, c, [], [], [], [], lb, ub, duty_cycles, options);
        
        % Update decay factor based on the current duty cycles
        [thrust_decay_factor, ~] = check_thrust_decay(duty_cycles);
                
        % Check convergence criteria
        if norm(duty_cycles - prev_duty_cycles, Inf) < tol
            H_final = MakeHWithDecayRecalculateForce(thruster_dist2CG_RED, F_red_X_nominal, thrust_decay_factor, F_red_Y_nominal);
            return;
        end
            
        
        % Update for next iteration
        prev_duty_cycles = duty_cycles;
    end
    
    H_final = MakeHWithDecayRecalculateForce(thruster_dist2CG_RED, F_red_X_nominal, thrust_decay_factor, F_red_Y_nominal);
   

end

function H = MakeHWithDecay(thruster_dist2CG, F_X_nominal, thrust_decay_factor, F_Y_nominal)
    % Constructs the H matrix with thrust decay adjustments
    %
    % Inputs:
    %   thruster_dist2CG - Distances of thrusters from CG (vector, mm)
    %   F_X_nominal - Nominal X thruster force (scalar, N)
    %   thrust_decay_factor - Decay factor for thrust (scalar)
    %   F_Y_nominal - Nominal Y thruster force (scalar, N)
    %
    % Output:
    %   H - H matrix for optimization (3x8)

    % Adjust thruster distances (convert to meters)
    adjusted_thruster_dist2CG = thruster_dist2CG / 1000;

    % Define thruster contribution vectors
    Vec1 = [-1; -1;  0;  0;  1;  1;  0;  0]; % X-component
    Vec2 = [ 0;  0;  1;  1;  0;  0; -1; -1]; % Y-component
    Vec3 = adjusted_thruster_dist2CG;        % Moment arm (Z)

    % Combine vectors into the H matrix structure
    Mat1 = [Vec1, Vec2, Vec3]';
    
    % Adjust thruster forces with decay factor
    F_thrusters = [F_X_nominal; F_X_nominal; F_Y_nominal; F_Y_nominal; 
                   F_X_nominal; F_X_nominal; F_Y_nominal; F_Y_nominal] * thrust_decay_factor;

    % Scale forces for H matrix
    Mat2 = diag(F_thrusters / 2);

    % Compute final H matrix
    H = Mat1 * Mat2;
end

function H = MakeHWithDecayRecalculateForce(thruster_dist2CG, F_X_nominal, thrust_decay_factor, F_Y_nominal)
    % Constructs the H matrix with thrust decay adjustments
    %
    % Inputs:
    %   thruster_dist2CG - Distances of thrusters from CG (vector, mm)
    %   F_X_nominal - Nominal X thruster force (scalar, N)
    %   thrust_decay_factor - Decay factor for thrust (scalar)
    %   F_Y_nominal - Nominal Y thruster force (scalar, N)
    %
    % Output:
    %   H - H matrix for optimization (3x8)

    % Adjust thruster distances (convert to meters)
    adjusted_thruster_dist2CG = thruster_dist2CG / 1000;

    % Define thruster contribution vectors
    Vec1 = [-1; -1;  0;  0;  1;  1;  0;  0]; % X-component
    Vec2 = [ 0;  0;  1;  1;  0;  0; -1; -1]; % Y-component
    Vec3 = adjusted_thruster_dist2CG;        % Moment arm (Z)

    % Combine vectors into the H matrix structure
    Mat1 = [Vec1, Vec2, Vec3]';
    
    % Adjust thruster forces with decay factor
    F_thrusters = [F_X_nominal; F_X_nominal; F_Y_nominal; F_Y_nominal; 
                   F_X_nominal; F_X_nominal; F_Y_nominal; F_Y_nominal] * thrust_decay_factor;

    % Scale forces for H matrix
    Mat2 = diag(F_thrusters);

    % Compute final H matrix
    H = Mat1 * Mat2;
end

function [thrust_decay_factor, count] = check_thrust_decay(PWMs)
    % Updates the thrust decay factor based on current duty cycles
    %
    % Inputs:
    %   PWMs - Current duty cycle values (vector)
    %
    % Outputs:
    %   thrust_decay_factor - Updated decay factor (scalar)
    %   count - Number of active thrusters (scalar)

    % Normalize PWMs if necessary
    if max(PWMs) > 1
        PWMs = PWMs / max(PWMs);
    end

    % Count active thrusters
    count = sum(PWMs > 0);
    
    % Compute average duty cycle for active thrusters
    average_duty_cycle_per_thruster = sum(max(PWMs, 0)) / max(count, 1);

    % Update thrust decay factor based on average duty cycle
    if average_duty_cycle_per_thruster < 0.3 || count == 0
        thrust_decay_factor = 1;
    else
        thrust_decay_factor = max(0.6 - 2 * average_duty_cycle_per_thruster + 1, 0.5);
    end
end

== matlab function MPC/Thruster Control Code/Change RED Behavior/Calculate Duty Cycle/MATLAB Function8 ==
  data: ThrustPer_Final output; ThrustPer input; PWMFreq parameter
function ThrustPer_Final  = ThrusterSat(ThrustPer, PWMFreq)

    ValveTime       = 0.007;
    TControl        = 1/PWMFreq;

    ThrustPer_Final = zeros(8,1);
    
    if max(ThrustPer) > 1
        ThrustPer_Sat = ThrustPer/max(ThrustPer);
    else
        ThrustPer_Sat = ThrustPer;
    end
    
    for i = 1:8
        if ThrustPer_Sat(i) > ValveTime/TControl 
            ThrustPer_Final(i) = ThrustPer_Sat(i);
        else
            ThrustPer_Final(i) = 0;
        end
    end


end

== matlab function MPC/Thruster Control Code/Change RED Behavior/Calculate Duty Cycle/Rotate Forces to Inertial/Create Rotation Matrix ==
  data: Rz input; C_Ib output
function C_Ib = RotateFrame(Rz)

C_bI = [  cos(Rz) sin(Rz)
         -sin(Rz) cos(Rz) ];

C_Ib = inv(C_bI);

end

== matlab function MPC/Thruster Control Code/Change RED Behavior/Rotate Forces to Body/Create Rotation Matrix ==
  data: Rz input; C_bI output
function C_bI = RotateFrame(Rz)

C_bI = [  cos(Rz) sin(Rz)
         -sin(Rz) cos(Rz) ];

end

== matlab function MPC/2 - Guidance/Custom PPL (BLACK)/Desired Position/MATLAB Function ==
  data: p0 input; pos_des output; pf input; duration input; t input
function pos_des = interpTrajectory(p0, pf, duration, t)
% interpTrajectory  Desired state along a straight‐line + constant spin
%
%   pos_des = interpTrajectory(p0, pf, duration, t) returns the desired
%   [x; y; theta] at time t, given:
%     p0       – [x0; y0; theta0]    initial position (m, m, rad)
%     pf       – [xf; yf; thetaf]    final position (m, m, rad) (thetaf unused)
%     duration – total time to go from p0 to pf (s)
%     t        – current time (s)
%
%   The (x,y) path is a straight line from p0 to pf over 'duration' seconds.
%   The yaw θ spins at a constant rate of 2π rad/60 s (1 rev/min), starting
%   from theta0.  If t<0 or t>duration, x,y are clamped to the endpoints.

  %--- clamp t into [0, duration]
  t_clamped = max(0, min(t, duration));

  %--- linear interpolation factor (0→1)
  s = t_clamped / duration;

  %--- interpolate x, y
  x_des = p0(1) + s*(pf(1) - p0(1));
  y_des = p0(2) + s*(pf(2) - p0(2));

  %--- constant angular rate: 1 rev/min = 2π/60 rad/s
  omega = 2*pi/60;
  omega = omega/4; % 60 was too fast
  theta_des = p0(3) + omega * t_clamped;

  %--- wrap angle into [0,2π)
  theta_des = mod(theta_des, 2*pi);

  %--- output as column vector
  pos_des = [x_des; y_des; theta_des];
end

== matlab function MPC/4 - Control/Default LQR Control (BLACK)/Calculate Error/MATLAB Function ==
  data: Rz_path input; Rz_error output; Rz_measured input
function Rz_error = SmoothAngularDifference(Rz_path, Rz_measured)

    Rz_error = mod(Rz_measured-Rz_path+pi, 2*pi)-pi;


end

== matlab function MPC/Data Logger Subsystem/Subsystem3/MATLAB Function ==
  data: u input; y output
function y = fcn(u)

if anynan(u)
    y = -1*ones(size(u));
else
    y = u;
end
end

== matlab function MPC/3 - Navigation/Subsystem/STDQMEKF1/MATLAB Function1 ==
  data: dt input; RED_dq input; VIS_dq input; x_est output; x_prev input; P_prev input; P_est output; compT output; y output; NIS output; V_prev input; V_est output
function [x_est, P_est, compT, y, NIS, V_est] = STDQMEKF(dt, RED_dq, VIS_dq, x_prev, P_prev, V_prev)

s1 = 1e-6;
s2 = 1e-6;
s3 = 1e-10;
s4 = 1e-7 ;
s5 = 0.06;
s6 = 0.001 ;
s7 = s6;

d1 = 1.6046;
d2 = 5.5866;

Q = blkdiag(s1*eye(3), s3*eye(3), s2*eye(3), s4*eye(3));


R = blkdiag(s5*eye(3), s6, s7*eye(2));

rho = 0.98;

maxd = [d1
        d2];

r = 0;
z = VIS_dq;
Chaser = RED_dq;

tic
[x_est, P_est, y, H, V_est] = runSTDQMEKF2(z, dt, ...
       x_prev, P_prev, Q, R, V_prev, r, rho, maxd, Chaser);
compT = toc;

Pzz = H*P_est*H' + R;
NIS = y' / Pzz * y;
end

== matlab function MPC/Data Logger Subsystem/Subsystem4/MATLAB Function ==
  data: u input; y output
function y = fcn(u)

if anynan(u)
    y = -1*ones(size(u));
else
    y = u;
end
end

== matlab function MPC/3 - Navigation/Subsystem/STDQMEKF1/MATLAB Function3 ==
  data: u input; x output
function x = fcn(u)
dq = [u(1:4),u(5:8)];
dv = [[0; u(9:11)], [0; u(12:14)]];
if norm(dq(:,1)) == 0
    dq = zeros(4,2);
    dq(1,1) = 1;
end
[q,r] = dq2quat(dq,'scalarFirst');
q = smallQuat(q,'scalarFirst');
v = dqLinearVelocity(dv, dq);
w = dv(2:4,1);
x = [q; r'; -w; -v];
end

function v_world = dqLinearVelocity(dq_vel, dq_pose)


    %-- 1) body‐frame linear velocity (pure quaternion) --%
    % Conjugate of the pose rotation quaternion:
    q_r_conj = quatConj(dq_pose(:,1),'scalarFirst');
    
    % pure‐quat v_body_q = 2 * (qv_dual * conj(q_pose.r))
    v_body_quat = 2 * quatMultiply(dq_vel(:,2), q_r_conj,'scalarFirst');
    
    %-- 2) rotate into world frame --%
    % dqRotate(q, p) ≡ q * p * conj(q) v_body_quat(2:4)
    v_world_quat = quatRotate(dq_pose(:,1), v_body_quat(2:4),'scalarFirst');
    
    %-- 3) extract vector part --%
    v_world = v_world_quat;

end

== matlab function MPC/3 - Navigation/Subsystem/STQMEKF1/MATLAB Function1 ==
  data: dt input; RED_quat input; RED_x input; BLACK_q input; BLACK_x input; x_est output; x_prev input; P_prev input; P_est output; compT output; y output; NIS output; V_prev input; V_est output; Q parameter; R parameter; maxd parameter; rho parameter
function [x_est, P_est, compT, y, NIS, V_est] = QMEKF(dt, RED_quat, RED_x, BLACK_q, BLACK_x, x_prev, P_prev, V_prev, Q, R, maxd, rho)

%% Best QMEKF values
s1 = 1e-6;
s2 = 1e-6;
s3 = 1e-10;
s4 = 1e-7 ;
s5 = 0.06;
s6 = 0.001 ;
s7 = s6;

d1 = 1.6046;
d2 = 5.5866;
rho = 0.98;

Q = blkdiag(s1*eye(3), s2*eye(3), s3*eye(3), s4*eye(3));


R = blkdiag(s5*eye(3), s6, s7*eye(2));

maxd = [d1
        d2];

%%
r = 0;
z = [BLACK_q; BLACK_x];
Chaser = [RED_quat; RED_x];

tic
[y, H, x_est, P_est, V_est] = runSTQMEKF2(z, dt, Chaser, ...
       x_prev, P_prev, V_prev, Q, R, r, rho, maxd);
compT = toc;

% Assume H is the full measurement matrix
S_att = H * P_est * H' + R;
NIS = y' / S_att * y;
end

== matlab function MPC/4 - Control/Default PD Control (RED)/CSMC/MATLAB Function2 ==
  data: q1 input; phi output; k1 parameter; alpha parameter; q2 input
function phi = fcn(q1,k1, alpha, q2)



phi = k1*q1 + (1/(2 - alpha))*sign(k1*q2)*(abs(k1*q2))^(2 - alpha);

== matlab function MPC/Simulate Plant Dynamics/RED and ARM Dynamics/RED + ARM/Dynamics Model ==
  data: q_dot output; x input; InertiaS input; CoriolisS input; u input; Gamma1_sh parameter; Gamma2_sh parameter; Gamma3_sh parameter; Gamma5_sh parameter; Gamma4_sh parameter; Gamma6_sh parameter; Gamma1_el parameter; Gamma2_el parameter; Gamma3_el parameter; Gamma5_el parameter; Gamma4_el parameter; Gamma6_el parameter; Gamma1_wr parameter; Gamma2_wr parameter; Gamma3_wr parameter; Gamma5_wr parameter; Gamma4_wr parameter; Gamma6_wr parameter; q_ddot output
function [q_dot, q_ddot]  = DynamicsModel(x, InertiaS, CoriolisS, u,...
    Gamma1_sh, Gamma2_sh, Gamma3_sh, Gamma5_sh, Gamma4_sh, Gamma6_sh,...
    Gamma1_el, Gamma2_el, Gamma3_el, Gamma5_el, Gamma4_el, Gamma6_el,...
    Gamma1_wr, Gamma2_wr, Gamma3_wr, Gamma5_wr, Gamma4_wr, Gamma6_wr)


    fqdot1 = Gamma1_sh*(tanh(Gamma2_sh*x(10)) - tanh(Gamma3_sh*x(10))) + Gamma4_sh*tanh(Gamma5_sh*x(10)) + Gamma6_sh*x(10);

    fqdot2 = Gamma1_el*(tanh(Gamma2_el*x(11)) - tanh(Gamma3_el*x(11))) + Gamma4_el*tanh(Gamma5_el*x(11)) + Gamma6_el*x(11);

    fqdot3 = Gamma1_wr*(tanh(Gamma2_wr*x(12)) - tanh(Gamma3_wr*x(12))) + Gamma4_wr*tanh(Gamma5_wr*x(12)) + Gamma6_wr*x(12);
    
    q_dot  = x(7:12);
    q_ddot = pinv(InertiaS)*(u - CoriolisS*x(7:12) - [0;0;0;fqdot1;fqdot2;fqdot3]);
    
end

== matlab function MPC/PhaseSpace Filter Code/Subsystem2/MATLAB Function ==
  data: dt input; z input; x output; P output; u input; x input; P input; V input; mBLACK parameter; IBLACK parameter; V output
function [x, P,V] = fcn(dt, z, u, x, P, V, mBLACK, IBLACK)
Q = blkdiag(0.0001*eye(2), 0.0000001);
R = 0.0000001*eye(3);
rho = 0.995;
Fargs.m = mBLACK;
Fargs.I = IBLACK;

% --- PREDICT ---------------------------------------------------------
[xk, F, G] = dyn(x,  dt, u, Fargs);
Pk         = F*P*F' + G*Q*G';

% --- For no Measurments ----------------------------------------------
if ~isfinite(z)
    x = xk;
    P = Pk;
    return
end

% --- Measurement -----------------------------------------------------
[zPred, H] = meas(xk, []);
y          = z - zPred;

% --- Angle Innovation (wrapped difference) ---------------------------
y(3) =  attErr(z(3),zPred(3));

% --- Strong Tracking -------------------------------------------------
% if det(V) == 0
%     V = rho*y*y';
% else
%     V = rho*(rho*V + y*y') / (1 + rho);
% end
% 
% L = corrP4Q(Pk, H, R, V);
% Pk = L*Pk*L';

% --- UPDATE ----------------------------------------------------------
S          = H*Pk*H' + R;
K          = Pk* H' / S;

corr       = K*y;
x          = xk + corr;
I          = eye(size(K,1));
P          = (I - K*H)*Pk*(I - K*H)' + K*R*K';

end

function [x,F,G] = dyn(x, dt, u, Fargs)
    F = [eye(3), dt*eye(3);
         zeros(3), eye(3)];

    m = diag([1/Fargs.m; 1/Fargs.m; 1/Fargs.I]);

    G = [(dt^2/2)*m; dt*m];

    x = F*x + G*u;
end

function [z, H] = meas(x, hargs)
    % H = eye(6);
    H = [eye(3), zeros(3)];
    z = H*x;
end

function e_out = attErr(ref,act)
Ax = [cos(act) sin(act); -sin(act) cos(act)]*[1;0];
Rx = [cos(ref) sin(ref); -sin(ref) cos(ref)]*[1;0];
Ry = [cos(ref) sin(ref); -sin(ref) cos(ref)]*[0;1];

e_in = Rx - Ax;

a = sign(Ry'*e_in);
e_out = -a*norm(e_in);
end

function L = corrP4Q(P_k, H, R, V)
    % Inputs:
    % P_K    - Time Updated Covar
    % H      - Measurement Jacobian
    % R      - Measurement covar
    % V      - True Pzz
    %
    % Find lambda Matrix
    % Initial guess for Lambda
    n = length(P_k);
    Lambda0 = ones(n/2,1); % Starting with an identity scaled by 2

    % Solve using Levenberg-Marquardt
    options = optimoptions('lsqnonlin', 'Algorithm', 'levenberg-marquardt','display','off');
    lb = ones(n/2,1);
    % Call lsqnonlin.
    Lambda_sol = lsqnonlin(@(x) objFun(x, eye(3), P_k, H, R, V), Lambda0, lb, [], options);
    L = blkdiag(diag(Lambda_sol(1:3)), ...
                     diag(Lambda_sol(1:3)));
end

function res = objFun(diagLambda, Izz, P, H, R, V)
    % Convert the vector of diagonal entries into a diagonal matrix Lambda.
    Lambda = blkdiag(diag(diagLambda(1:3)), ...
                     diag(diagLambda(1:3)));
    
    % Update the state covariance using the matrix fading factor.
    P_new = Lambda * P * Lambda;
    
    % Compute the measurement covariance.
    Pzz = H * P_new * H' + R;
    
    % Compute the residual. The goal is to have Pzz^{-1} * V as close as possible
    % to the identity Izz.
    % (Depending on your filter design, you may have a different function to minimize.)
    resMat = Izz - inv(Pzz) * V;
    
    % Return the residual as a vector (by stacking the matrix columns).
    res = resMat(:);
end

== matlab function MPC/4 - Control/Default PD Control (RED)/CSMC/MATLAB Function3 ==
  data: phi input; u output; alpha parameter
function u = fcn(phi, alpha)



u = sign(phi)*(abs(phi)^(alpha/(2 - alpha)));
